simulink model "fp_arith_denormalize"  (Simulink 7.6)
settings: Solver=FixedStepDiscrete  StartTime=0.0  StopTime=10.0  FixedStep=1  RelTol=1e-3
settings Model: Creator=jordan  LastModifiedBy=jordan
settings DataIOCC: LimitDataPoints=off  SaveOutput=off  SignalLogging=off  DSMLogging=off  SaveTime=off
settings OptimizationCC: BlockReduction=off  ConditionallyExecuteInputs=off

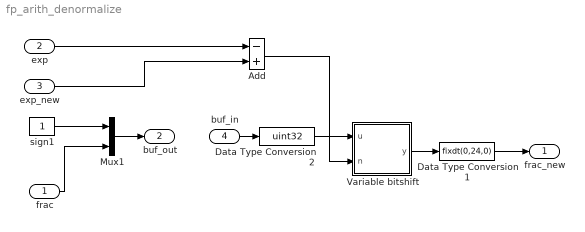
== system fp_arith_denormalize ==
  frac : Inport  OutDataTypeStr=boolean  PortDimensions=23
  exp : Inport  Port=2  OutDataTypeStr=uint8
  exp_new : Inport  Port=3  OutDataTypeStr=uint8
  buf_in : Inport  Port=4  OutDataTypeStr=fixdt(0,24,0)
  Add : Sum  Inputs=-+  OutDataTypeStr=int8
  Data Type Conversion1 : DataTypeConversion  OutDataTypeStr=fixdt(0,24,0)
  Data Type Conversion2 : DataTypeConversion  OutDataTypeStr=uint32
  Mux1 : Mux  Inputs=2
  Variable bitshift : Stateflow chart  TreatAsAtomicUnit=on
  sign1 : Constant  OutDataTypeStr=boolean
  frac_new : Outport
  buf_out : Outport  Port=2  OutDataTypeStr=boolean  PortDimensions=24
  wires:
  frac/1 -> Mux1/2
  Add/1 -> Variable bitshift/2(n)
  Mux1/1 -> buf_out/1
  sign1/1 -> Mux1/1
  buf_in/1 -> Data Type Conversion2/1
  Variable bitshift/1(y) -> Data Type Conversion1/1
  exp/1 -> Add/1
  exp_new/1 -> Add/2
  Data Type Conversion1/1 -> frac_new/1
  Data Type Conversion2/1 -> Variable bitshift/1(u)

== matlab function Variable bitshift ==
  data: u input uint32; y output uint32; n input int8
function y = fcn(u,n)
%#eml

y = bitshift(u,-n);
